simulink model "flatness_temp"  (R2024b)
settings: Solver=ode4  StartTime=0  StopTime=100  FixedStep=1e-2  RelTol=1e-3  AbsTol=1e-6
libraries: vrlib x1
settings Model: Creator=jerome  LastModifiedBy=therkelsen
settings SolverCC: AutoScaleAbsTol=off  AlgebraicLoopSolver=TrustRegion
settings DataIOCC: SaveFormat=Array  SignalLoggingSaveFormat=ModelDataLogs  ReturnWorkspaceOutputs=off
settings OptimizationCC: BlockReduction=off  BooleanDataType=off  ExpressionDepthLimit=2147483647  InitFltsAndDblsToZero=on  LifeSpan=inf
settings DebuggingCC: SaveWithParameterizedLinksMsg=none  UnderspecifiedInitializationDetection=Classic  MergeDetectMultiDrivingBlocksExec=none  SignalResolutionControl=TryResolveAllWithWarning  MultiTaskDSMMsg=warning  MultiTaskCondExecSysMsg=none  FcnCallInpInsideContextMsg=warning  UnconnectedInputMsg=warning  UnconnectedOutputMsg=warning  UnconnectedLineMsg=warning  StateNameClashWarn=warning  SFUnexpectedBacktrackingDiag=warning  SFNoUnconditionalDefaultTransitionDiag=warning  SFExecutionAtInitializationDiag=none  ArithmeticOperatorsInVariantConditions=warning
settings HardwareCC: ProdBitPerPointer=32  ProdBitPerSizeT=32  ProdBitPerPtrDiffT=32  ProdLargestAtomicFloat=None  ProdIntDivRoundTo=Undefined  ProdEndianess=Unspecified  ProdWordSize=32  ProdHWDeviceType=32-bit Generic  TargetUnknown=on
settings ModelReferenceCC: EnableRefExpFcnMdlSchedulingChecks=on  PropagateSignalLabelsOutOfModel=off
settings SFSimCC: SimUseLocalCustomCode=off  CustomCodeUndefinedFunction=UseInterfaceOnly
settings RTWCC: RTWUseLocalCustomCode=off  GPUComputeCapability=3.5  DLArmComputeVersion=19.05
settings CodeAppCC: StateflowObjectComments=on
settings GRTTargetCC: TargetFcnLib=ansi_tfl_tmw.mat  TargetLangStandard=C89/C90 (ANSI)  ModelReferenceCompliant=off  CombineOutputUpdateFcns=off  MatFileLogging=off  GRTInterface=on
settings ConfigComp: CovMetricSettings=dw  CovSaveCumulativeToWorkspaceVar=on  CovSaveSingleToWorkspaceVar=on  CovExternalEMLEnable=off

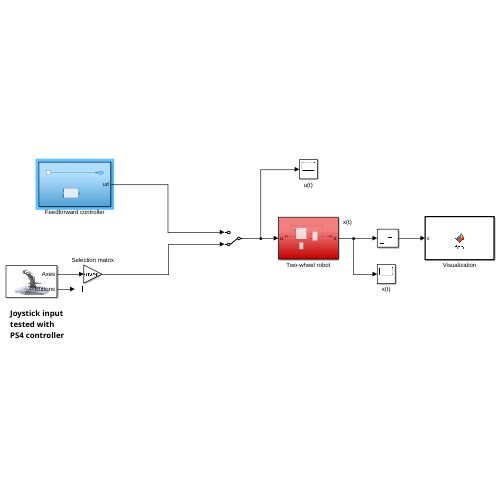
[thumbnail: Simulink's stored preview of the top-level diagram]
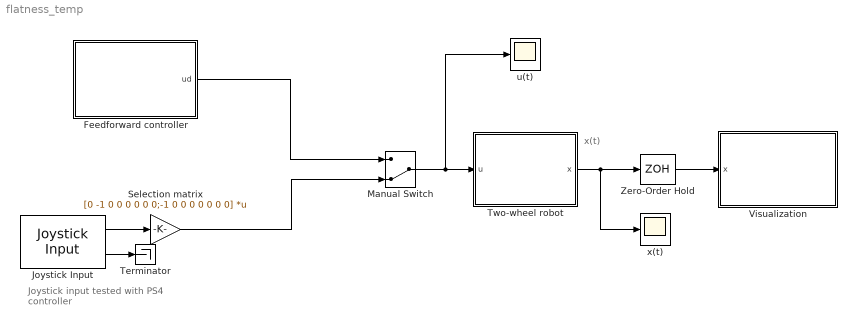
== system flatness_temp ==
  note: Joystick input
      | tested with
      | PS4 controller
  note: x(t)
  Feedforward controller : Subsystem
  Joystick Input : vrlib/Joystick Input  joyid=1  adjustports=off  forcefeed=off
  Manual Switch : ManualSwitch  CurrentSetting=0
  Selection matrix : Gain  Gain=[0 -1 0 0 0 0 0 0;-1 0 0 0 0 0 0 0]  Multiplication=Matrix(K*u) (u vector)
  Terminator : Terminator
  Two-wheel robot : Subsystem
  Visualization : MATLAB Function  TreatAsAtomicUnit=on
  Zero-Order Hold : ZeroOrderHold  SampleTime=0.1
  u(t) : Scope
  x(t) : Scope
  wires:
  Joystick Input/2 -> Terminator/1
  Joystick Input/1 -> Selection matrix/1
  Zero-Order Hold/1 -> Visualization/1(x)
  Two-wheel robot/1(x) -> x(t)/1, Zero-Order Hold/1
  Manual Switch/1 -> u(t)/1, Two-wheel robot/1(u)
  Selection matrix/1 -> Manual Switch/2
  Feedforward controller/1(ud) -> Manual Switch/1

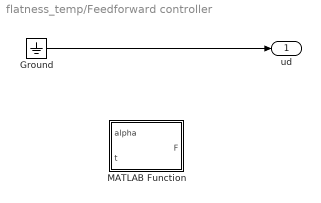
== system flatness_temp/Feedforward controller ==
  Ground : Ground
  MATLAB Function : MATLAB Function  TreatAsAtomicUnit=on
  ud : Outport
  wires:
  Ground/1 -> ud/1

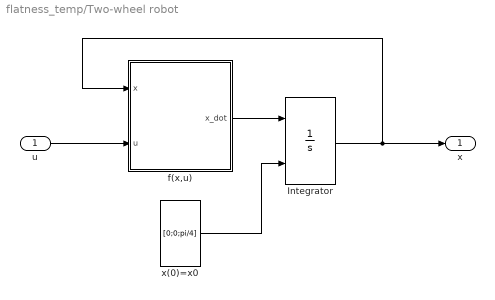
== system flatness_temp/Two-wheel robot ==
  u : Inport
  Integrator : Integrator  InitialConditionSource=external
  f(x,u) : MATLAB Function  TreatAsAtomicUnit=on
  x(0)=x0 : Constant  Value=[0;0;pi/4]  VectorParams1D=off
  x : Outport
  wires:
  u/1 -> f(x,u)/2(u)
  x(0)=x0/1 -> Integrator/2
  Integrator/1 -> x/1, f(x,u)/1(x)
  f(x,u)/1(x_dot) -> Integrator/1

== matlab function flatness_temp/Two-wheel robot/f(x,u) ==
  data: x input; u input; x_dot output
function x_dot = f(x,u)

% dynamic variables
x1 = x(1);
x2 = x(2);
theta = x(3);

% control inputs
u1 = u(1);
u2 = u(2);

x1_dot = u1*cos(theta);
x2_dot = u1*sin(theta);
theta_dot = u2;

x_dot = [ x1_dot ; x2_dot ; theta_dot ];

== matlab function flatness_temp/Feedforward controller/MATLAB Function ==
  data: alpha input; t input; F output
function F = flat_outputs(alpha, t)

== matlab function flatness_temp/Visualization ==
  data: x input
function fcn(x)

x1 = x(1);
x2 = x(2);
theta = x(3);

% body "shape"
    Ybody = [ -0.2 ; -0.2 ; 0.2 ; 0.2 ];
    Xbody = [ -0.15 ; 0.15 ; 0.15 ; -0.15 ]; 

% front "shape" 
    Yfront = [ -0.2 ; -0.1 ; 0.1 ; 0.2 ];
    Xfront = [ 0.15 ; 0.2 ; 0.2 ; 0.15 ];
    
% wheel model "shape"
    Yw = [ -0.02 ; -0.02 ; 0.02 ; 0.02 ];
    Xw = [ -0.13 ; 0.13 ; 0.13 ; -0.13 ];
    
% left wheel
    Ywl = Yw + 0.21;
    Xwl = Xw;
    
% right wheel    
    Ywr = Yw - 0.21;
    Xwr = Xw;

% rotation and translation of 2-wheel robot body

[PosXbody,PosYbody] = rot(Xbody,Ybody,theta);
PosXbody = PosXbody + x1;
PosYbody = PosYbody + x2;
[PosXwl,PosYwl] = rot(Xwl,Ywl,theta);
PosXwl = PosXwl + x1;
PosYwl = PosYwl + x2;
[PosXwr,PosYwr] = rot(Xwr,Ywr,theta);
PosXwr = PosXwr + x1;
PosYwr = PosYwr + x2;
[PosXfront,PosYfront] = rot(Xfront,Yfront,theta);
PosXfront = PosXfront + x1;
PosYfront = PosYfront + x2;

% to be able to use 'fill' even though the function is not supported for code generation
% see https://se.mathworks.com/help/simulink/slref/coder.extrinsic.html
coder.extrinsic('fill'); 

% draw body and put colors in
fill(PosXbody,PosYbody,'r',PosXwl,PosYwl,'b',PosXwr,PosYwr,'b',PosXfront,PosYfront,'g');

axis([-1 6 -1 6]);
title('2-wheeled robot');
grid on;
drawnow;



% function "rot" that rotates a graphical object
function [PosX,PosY] = rot(X,Y,angle)

dim1 = size(X,1);
dim2 = size(X,2);
PosX = zeros(dim1,dim2);
PosY = zeros(dim1,dim2);

Mrot = [ cos(angle) -sin(angle)  ;
         sin(angle)  cos(angle) ]; 

for i=1:dim1
    Pos_i = Mrot * [ X(i,1) ; Y(i,1) ];
    PosX(i,1) = Pos_i(1,1);
    PosY(i,1) = Pos_i(2,1);
end
